simulink model "RHONN_EKF_FEEDBACK_FINAL_28_JULIO_2021"  (R2017b)
settings: Solver=ode1  StartTime=0.0  StopTime=60  FixedStep=0.001  RelTol=1e-3
model workspace (MATLAB code in the model file):
  | % ESTADOS INICIALES DE LOS ESTADOS X1, X2 Y X3
  | % Donde:
  | % x1 es representado con un vector de 3x1.
  | % x2 es representado con un vector de 2x1.
  | % x3 es representado con un vector de 2x1.
  | 
  | % Definir estados iniciales de las variables x11, x12 y x13 respectivamente.
  | init_x11 = 0;
  | init_x12 = 0;
  | init_x13 = 0;
  | % Estado inicial de x1
  | init_state_x1 = [init_x11; init_x12; init_x13];
  | 
  | % Definir estados iniciales de las variables x21 y x22 respectivamente.
  | init_x21 = 0.1;
  | init_x22 = 0.1;
  | % Estado inicial de x2
  | init_state_x2 = [init_x21; init_x22];
  | 
  | % Definir estados iniciales de las variables x31 y x32 respectivamente.
  | init_x31 = 0.1;
  | init_x32 = 0.1;
  | % Estado inicial de x3
  | init_state_x3 = [init_x31; init_x32];
  | 
  | % Definir el estado inicial de la ley de control U, representado por un vector de 2x1.
  | init_U1 = -1;
  | init_U2 = -1;
  | init_U = [init_U1; init_U2];
  | 
  | % INICIALIZACION DE VARIABLES >>>>>>>>>>>>>>>>>>>>>>>>>>>>>>>>
  | 
  |     %Constantes iniciales
  |     %La mitad del ancho del robot mobil.
  |     R = 0.75;
  |     %La distancia del centro de Pc del robot mobil a la mitad del punto medio
  |     %de P0 en medio de las ruedas izquierda y derecha.
  |     d = 0.3;
  |     %Radio de la rueda.
  |     r = 0.15;
  |     %Masa del cuerpo.
  |     mc = 30;
  |     %Masa de la rueda con motor.
  |     mw = 1;
  |     %Ic,Iw,Im son los momentos de inercia del cuerpo sobre el eje vertical a
  |     %traves de Pc.
  |     Ic = 15.625;
  |     Iw = 0.005;
  |     Im = 0.0025;
  |     %Resistencia.
  |     Ra = diag([2.5,2.5]);
  |     %Inductancia.
  |     La = diag([0.048,0.048]);
  |     %Coeficiente de fuera electromotriz trasero.
  |     KE = diag([0.02,0.02]);
  |     %Relacion de transmision.
  |     N = diag([62.55,62.55]);
  |     %Constante de torque del motor.
  |     KT = diag([0.2613,0.2613]);
  |     %d11, d12 son los coeficientes de amortiguamiento.
  |     d11 = 0.5;
  |     d12 = d11;
  |     %>>>>>>>>>>>>>>>>>>>>>>>>>>>>>>>>>>>>>>>>>>>>>>>>>>>>>>>><
  | 
  |     m = mc + (2 * mw);
  |     I = (mc * (d ^ 2)) + (2 * mw * (R^2)) + Ic + (2*Im);
  |     m11 = 0.25 * ( R ^ -2 ) * (r ^ 2) * ((m * (R ^ 2)) + I) + Iw;
  |     m12 = 0.25 * ( R ^ -2 ) * (r ^ 2) * ((m * (R ^ 2)) - I);
  |     M = [m11, m12; m12, m11];
  |     D = diag([d11, d12]);
  | 
  | 
  |  %VALORES HUERISTICOS SEGUN EL PAPER
  | %MODELO MATEMATICO
  | 
  | 
  | %Constantes iniciales
  | %La mitad del ancho del robot mobil.
  | R = 0.75;
  | %La distancia del centro de Pc del robot mobil a la mitad del punto medio
  | %de P0 en medio de las ruedas izquierda y derecha.
  | d = 0.3;
  | %Radio de la rueda.
  | r = 0.15;
  | %Masa del cuerpo.
  | mc = 30;
  | %Masa de la rueda con motor.
  | mw = 1;
  | %Ic,Iw,Im son los momentos de inercia del cuerpo sobre el eje vertical a
  | %traves de Pc.
  | Ic = 15.625;
  | Iw = 0.005;
  | Im = 0.0025;
  | %Resistencia.
  | Ra = diag([2.5,2.5]);
  | %Inductancia.
  | La = diag([0.048,0.048]);
  | %Coeficiente de fuera electromotriz trasero.
  | KE = diag([0.02,0.02]);
  | %Relacion de transmision.
  | N = diag([62.55,62.55]);
  | %Constante de torque del motor.
  | KT = diag([0.2613,0.2613]);
  | %d11, d12 son los coeficientes de amortiguamiento.
  | d11 = 0.5;
  | d12 = d11;
  | 
  | 
  | 
  | %NOTA : los valores cuya definicion se encuentre en minuscula
  | %se utiliza para generar de manera dinamica con programacion
  | %la variable final que se utiliza en el programa.
  | %De manera que si llegara a ser necesario solo se modificarian las variables iniciales
  | 
  | %VARIABLES INICIALES ========================================
  | 
  | p1 = 1 * (10^8);
  | p2 = 1 * (10^2);
  | p3 = 1 * (10^8);
  | p4 = 1 * (10^2);
  | p5 = 1 * (10^2);
  | p6 = 1 * (10^2);
  | p7 = 1 * (10^2);
  | 
  | r1 = 1 * (10^4);
  | r2 = 5 * (10^4);
  | r3 = 1 * (10^4);
  | r4 = 1 * (10^1);
  | r5 = 1 * (10^1);
  | r6 = 1 * (10^3);
  | r7 = 1 * (10^3);
  | 
  | q1 = 5 * (10^5);
  | q2 = 5 * (10^5);
  | q3 = 5 * (10^5);
  | q4 = 1 * (10^1);
  | q5 = 1 * (10^1);
  | q6 = 1 * (10^3);
  | q7 = 1 * (10^3);
  | 
  | G1 = 0.00001;
  | G2 = 0.00001;
  | 
  | %VALOREES INICIALES DE LOS PESOS USADOS EN EKF
  | 
  | %PESOS DE W1
  | W11 = 0.1;
  | W12 = 0.1;
  | %PESOS DE W2
  | W21 = 0.1;
  | W22 = 0.1;
  | %PESOS DE W3
  | W31 = 0.1;
  | W32 = 0.1;
  | %PESOS DE W4
  | W41 = 0.1;
  | W42 = 0.1;
  | W43 = 0.1;
  | W44 = 0.1;
  | %PESOS DE W5
  | W51 = 0.1;
  | W52 = 0.1;
  | W53 = 0.1;
  | W54 = 0.1;
  | %PESOS DE W6
  | W61 = 0.1;
  | W62 = 0.1;
  | W63 = 0.1;
  | W64 = 0.1;
  | %PESOS DE W7
  | W71 = 0.1;
  | W72 = 0.1;
  | W73 = 0.1;
  | W74 = 0.1;
  | 
  | %VALOR DE LAS SIGMOIDALES SUAVES
  | B = 2 * exp(-3);    %Este valor debe ser mayor a cero pero en base a mis observaciones menor a 1.
  | FO = 1;   %Este valor es obtenido de la tesis de la Dra Alma debe ser CERCANO y MENOR a 1, si este se vuelve 1 funcionara como FKE unicamente
  | 
  | 
  | %VARIABLES FINALES ========================================
  | 
  | %PARAMETROS DE ENTRENAMIENTO EKF PARA RHONN 1
  | W1 = [W11; W12]; %VALOR INICIAL de Vector de pesos para x1
  | P1 = diag([p1, p1]); %VALOR INICIAL de Matriz diagonal inicial de P1
  | R1 = r1; % Valor de R1
  | Q1 = diag([q1, q1]); % Valor de Q1
  | 
  | %PARAMETROS DE ENTRENAMIENTO EKF PARA RHONN 2
  | W2 = [W21; W22]; %VALOR INICIAL de Vector de pesos para x2
  | P2 = diag([p2, p2]); %VALOR INICIAL de Matriz diagonal inicial de P2
  | R2 = r2; % Valor de R2
  | Q2 = diag([q2, q2]); % Valor de Q2
  | 
  | %PARAMETROS DE ENTRENAMIENTO EKF PARA RHONN 3
  | W3 = [W31; W32]; %VALOR INICIAL de Vector de pesos para x3
  | P3 = diag([p3, p3]); %VALOR INICIAL de Matriz diagonal inicial de P3
  | R3 = r3; % Valor de R3
  | Q3 = diag([q3, q3]); % Valor de Q3
  | 
  | %PARAMETROS DE ENTRENAMIENTO EKF PARA RHONN 4
  | W4 = [W41; W42; W43; W44]; %VALOR INICIAL de Vector de pesos para x4
  | P4 = diag([p4, p4, p4, p4]); %VALOR INICIAL de Matriz diagonal inicial de P4
  | R4 = r4; % Valor de R4
  | Q4 = diag([q4, q4, q4, q4]); % Valor de Q4
  | 
  | %PARAMETROS DE ENTRENAMIENTO EKF PARA RHONN 5
  | W5 = [W51; W52; W53; W54]; %VALOR INICIAL de Vector de pesos para x5
  | P5 = diag([p5, p5, p5, p5]); %VALOR INICIAL de Matriz diagonal inicial de P5
  | R5 = r5; % Valor de R5
  | Q5 = diag([q5, q5, q5, q5]); % Valor de Q5
  | 
  | %PARAMETROS DE ENTRENAMIENTO EKF PARA RHONN 6
  | W6 = [W61; W62; W63; W64]; %VALOR INICIAL de Vector de pesos para x6
  | P6 = diag([p6, p6, p6, p6]); %VALOR INICIAL de Matriz diagonal inicial de P6
  | R6 = r6; % Valor de R6
  | Q6 = diag([q6, q6, q6, q6]); % Valor de Q6
  | 
  | %PARAMETROS DE ENTRENAMIENTO EKF PARA RHONN 7
  | W7 = [W71; W72; W73; W74]; %VALOR INICIAL de Vector de pesos para x7
  | P7 = diag([p7, p7, p7, p7]); %VALOR INICIAL de Matriz diagonal inicial de P7
  | R7 = r7; % Valor de R7
  | Q7 = diag([q7, q7, q7, q7]); % Valor de Q7
  | 
  | 
  | % PARAMETROS DEL CONTROL POR RETROALIMENTACION
  | % Donde K1 es representado con una matriz diagonal 3x3
  | % Donde K2 es representado con una matriz diagonal 2x2
  | % Donde K3 es representado con una matriz diagonal 2x2
  | 
  | % Ganancias individuales de la diagonal K1
  | k11 = 70;
  | k12 = k11;
  | k13 = k11;
  | 
  | % Ganancias individuales de la diagonal K2.
  | k21 = 50;
  | k22 = k21;
  | 
  | % Ganancias individuales de la diagonal K3.
  | k31 = 200;
  | k32 = k31;
  | 
  | % Matrices de gananciasK1, K2, K3.
  | K1 = diag([k11, k12, k13]);
  | K2 = diag([k21, k22]);
  | K3 = diag([k31, k32]);
libraries: simulink x5
(part 2 of 2)

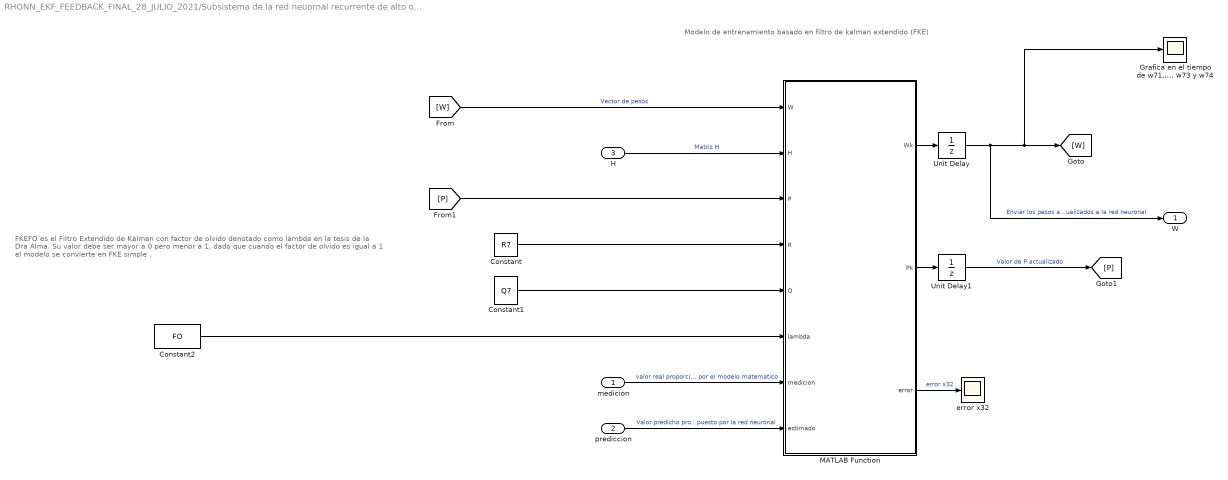
== system RHONN_EKF_FEEDBACK_FINAL_28_JULIO_2021/Subsistema de la red neuornal recurrente de alto orden (RHONN)/X7_RHONN/X7_EKF ==
  note: FKEFO es el Filtro Extendido de Kalman con factor de olvido
      |
      | denotado como lambda en la tesis de la Dra Alma.
      | Su valor debe ser mayor a 0 pero menor a 1, dado que cuando
      | el factor de olvido es igual a 1 el modelo se convierte en FKE simple .
  note: Modelo de entrenamiento basado en filtro de kalman extendido (FKE)
  medicion : Inport
  prediccion : Inport  Port=2
  H : Inport  Port=3
  Constant : Constant  Value=R7
  Constant1 : Constant  Value=Q7
  Constant2 : Constant  Value=FO
  "Grafica en el tiempo de w71, w72, w73 y w74" : Scope
  MATLAB Function : MATLAB Function  TreatAsAtomicUnit=on
  Unit Delay : UnitDelay  InitialCondition=W7  SampleTime=-1
  Unit Delay1 : UnitDelay  InitialCondition=P7  SampleTime=-1
  error x32 : Scope
  W : Outport
  wires:
  prediccion/1 -> MATLAB Function/8(estimado)  "Valor predicho propuesto por la red neuronal"
  medicion/1 -> MATLAB Function/7(medicion)  "valor real proporcionado por el modelo matematico"
  MATLAB Function/1(Wk) -> Unit Delay/1
  [W] -> MATLAB Function/1(W)  "Vector de pesos"
  MATLAB Function/2(Pk) -> Unit Delay1/1
  [P] -> MATLAB Function/3(P)
  Constant/1 -> MATLAB Function/4(R)
  Constant1/1 -> MATLAB Function/5(Q)
  H/1 -> MATLAB Function/2(H)  "Matriz H"
  Unit Delay1/1 -> [P]  "Valor de P actualizado"
  Unit Delay/1 -> "Grafica en el tiempo de w71, w72, w73 y w74"/1, [W], W/1  "Enviar los pesos actualizados a la red neuronal"
  Constant2/1 -> MATLAB Function/6(lambda)
  MATLAB Function/3(error) -> error x32/1  "error x32"

== matlab function RHONN_EKF_FEEDBACK_FINAL_28_JULIO_2021/Subsistema del robot no-holonomico, Modelo cinematico/NonHolonomic robot PLANT Function ==
  data: x11 input; dx1 output; x12 input; x13 input; dx13 input; x21 input; x22 input; x31 input; x32 input; Td1 input; Td2 input; dx2 output; dx3 output; u input
function [dx1,dx2,dx3]  = ROBOT(x11, x12, x13, dx13, x21, x22, x31, x32, Td1, Td2, u)
    
    %Definicion de las matrices de parametros del robot.(Entradas).
    x1 = [x11; x12; x13];
    x2 = [x21; x22];
    x3 = [x31; x32];
    
    %Vector de perturbaciones.
    Td = [Td1; Td2];
    
    %Vector de torques.
    %T = [T1; T2];
   
    %Vector de voltajes
    %u = [u1;u2];
    %Constantes iniciales
    %La mitad del ancho del robot mobil.
    R = 0.75;
    %La distancia del centro de Pc del robot mobil a la mitad del punto medio
    %de P0 en medio de las ruedas izquierda y derecha.
    d = 0.3;
    %Radio de la rueda.
    r = 0.15;
    %Masa del cuerpo.
    mc = 30;
    %Masa de la rueda con motor.
    mw = 1;
    %Ic,Iw,Im son los momentos de inercia del cuerpo sobre el eje vertical a
    %traves de Pc.
    Ic = 15.625;
    Iw = 0.005;
    Im = 0.0025;
    %Resistencia.
    Ra = diag([2.5,2.5]);
    %Inductancia.
    La = diag([0.048,0.048]);
    %Coeficiente de fuera electromotriz trasero.
    KE = diag([0.02,0.02]);
    %Relacion de transmision.
    N = diag([62.55,62.55]);
    %Constante de torque del motor.
    KT = diag([0.2613,0.2613]);
    %d11, d12 son los coeficientes de amortiguamiento.
    d11 = 0.5;
    d12 = d11;

    %%%%%%%%%%%%%% Constantes productos de otras constantes%%%%%%%%%%%%%%%%%%%%

    %Matriz cinematica del robot
    Jx1 = 0.5*r*[cos(x13), cos(x13); sin(x13), sin(x13); 1/R,-1/R];
    
    m = mc + (2 * mw);
    I = (mc * (d ^ 2)) + (2 * mw * (R^2)) + Ic + (2*Im);
    m11 = 0.25 * ( R ^ -2 ) * (r ^ 2) * ((m * (R ^ 2)) + I) + Iw;
    m12 = 0.25 * ( R ^ -2 ) * (r ^ 2) * ((m * (R ^ 2)) - I);
    M = [m11, m12; m12, m11];
    D = diag([d11, d12]);
    Cdx1 = 0.5*(1/R)*(r^2)*mc*d*[0, dx13; -dx13 0];
    
    %Definiendo las salidas de la funcion 
    dx1 = Jx1*x2;
    dx2=M\(-Cdx1*x2-D*x2-Td+(N*KT*x3));
    dx3 = La\(u-Ra*x3-(N*KE*x2));
    
    
end

== matlab function RHONN_EKF_FEEDBACK_FINAL_28_JULIO_2021/Trayectoria de referencia generada/Reference robot function ==
  data: Vr input; Wr input; dx1r output; Or input
function dx1r = fcn(Vr,Wr,Or)
    %   Definimos la señal de entrada que viene en el vector Zr' 
    dor = Wr;
    dxr = Vr * cos(Or);
    dyr = Vr * sin(Or);
    dx1r = [dxr; dyr; dor];

== matlab function RHONN_EKF_FEEDBACK_FINAL_28_JULIO_2021/Subsistema de la red neuornal recurrente de alto orden (RHONN)/X1_RHONN/Sigmoidal suave1/Sigmoidal suave ==
  data: B input; sig output; c input
function sig = fcn(B, c)

%Ecuacion sigmoidal suave
sig = 1/ (1 + exp(-B * c));

== matlab function RHONN_EKF_FEEDBACK_FINAL_28_JULIO_2021/Subsistema de la red neuornal recurrente de alto orden (RHONN)/X1_RHONN/Sigmoidal suave3/Sigmoidal suave ==
  data: B input; sig output; c input
function sig = fcn(B, c)

%Ecuacion sigmoidal suave
sig = 1/ (1 + exp(-B * c));

== matlab function RHONN_EKF_FEEDBACK_FINAL_28_JULIO_2021/Subsistema de la red neuornal recurrente de alto orden (RHONN)/X1_RHONN/X1_RHONN ==
  data: W input; pred output; Sx11 input; Sx12 input
function pred = fcn(W,Sx11,Sx12)
    
    %Pesos de la RHONN
    w11 = W(1);
    w12 = W(2);
    %Ecuacion de prediccion
    pred = ( w11 * Sx11 ) + ( w12 * Sx12 );

== matlab function RHONN_EKF_FEEDBACK_FINAL_28_JULIO_2021/Subsistema de control por retroalimentacion/MATLAB Function ==
  data: x1 input; x1r input; x2 input; dx1r input; x13 input; dx13 input; e1 output; e2 output; e3 output; U output; x3 input; k1 input; k2 input; k3 input
function [e1, e2, e3,U] = fcn(x1, x1r, x2,dx1r, x13, dx13, x3, k1, k2, k3)

   
    Td = [0.5; 0.5];
    %Constantes iniciales
    R = 0.75;    %La mitad del ancho del robot mobil.
    d = 0.3; %La distancia del centro de Pc del robot mobil a la mitad del punto medio
             %de P0 en medio de las ruedas izquierda y derecha
    r = 0.15; %Radio de la rueda.
    mc = 30;  %Masa del cuerpo.
    mw = 1;  %Masa de la rueda con motor.
    %Ic,Iw,Im son los momentos de inercia del cuerpo sobre el eje vertical a
    %traves de Pc.
    Ic = 15.625;
    Iw = 0.005;
    Im = 0.0025;
   
    Ra = diag([2.5,2.5]);       %Resistencia.
    La = diag([0.048,0.048]);    %Inductancia.
    KE = diag([0.02,0.02]);     %Coeficiente de fuera electromotriz trasero.
    N = diag([62.55,62.55]);     %Relacion de transmision.
    KT = diag([0.2613,0.2613]);  %Constante de torque del motor.
    d11 = 0.5;         %d11, d12 son los coeficientes de amortiguamiento.
    d12 = d11;

    m = mc + (2 * mw);
    I = (mc * (d ^ 2)) + (2 * mw * (R^2)) + Ic + (2*Im);
    m11 = 0.25 * ( R ^ -2 ) * (r ^ 2) * ((m * (R ^ 2)) + I) + Iw;
    m12 = 0.25 * ( R ^ -2 ) * (r ^ 2) * ((m * (R ^ 2)) - I);
    M = [m11, m12; m12, m11];
    D = diag([d11, d12]);
    Cdx1 = 0.5 * (1/R) * (r ^ 2) * mc * d * [0, dx13; -dx13 0];
    
    %%%%%%%%%%%%%%%%%%%%%%%%%%%%%%%%%%%%%%%%%%%%%%%%%%%%%%%%%%%%%%%%%%%%%%%
    
    % Control
    %Matriz cinematica del robot
     
    Jx1=0.5*r*[cos(x13), cos(x13); sin(x13), sin(x13); 1/R,-1/R];
    Jx1_inversa = pinv(Jx1);
	%Control virtual para x2r virtual.
    e1=x1-x1r;
    x2r=Jx1_inversa*(-k1*e1-dx1r);
    e2=x2-x2r;
    % Control virtual para x3r virual.
    dx2r = diff(x2r);
    x3r = (N*KT)\(M*(-k2*e2+dx2r)+Cdx1*x2+D*x2+Td);
    e3=x3-x3r;
    % Control real U.
    dx3r = diff(x3r);
    U=La*(-k3*e3+dx3r)+Ra*x3+N*KE*x2;
end

== matlab function RHONN_EKF_FEEDBACK_FINAL_28_JULIO_2021/Subsistema de la red neuornal recurrente de alto orden (RHONN)/X1_RHONN/X1_EKF/MATLAB Function ==
  settings: updateMethod=DISCRETE
  data: W input; Wk output; H input; P input; R input; Q input; lambda input; medicion input; estimado input; Pk output; error output
function [Wk, Pk, error] = fcn(W, H, P, R, Q, lambda, medicion, estimado)
    % Se inicializan las dimenciones de las variables K y M para evitar
    % error de dimensiones al momento de compilar.
    persistent K
    persistent M
    
    if isempty(K)
        K = zeros(2,1);
    end
    
    if isempty(M)
        M = zeros(1,1);
    end
    
    % NOTA: Para este caso
    % W, H, P, R, Q representan los valores en k_esima
    % Wk, Pk representan los valores de k + 1
    
    %L es el numero total de pesos = 2 (w11,w12)
    %m es el numero de salidas = 1 (X(k+1))
    
    %P es una matriz L x L (2x2)
    %R es una matriz m x m (1x1)
    %Q es una matriz L x L (2x2)
    %K es una matriz L x m (2x1)
    
    %lambda es el factor de olvido si lambda = 1 el modelo deja de ser
    %FKEFO y se vuelve FKE
    error = medicion - estimado;
    %Mi(k)
    M = (R * lambda ) + (H * P * H');
    %K(k)
    K = (P * H' )/(M);
    %W(k+1)
    Wk = W + K * (medicion - estimado);
    %P(k+1)
    Pk = (P * (1/lambda)) - ((1/lambda) * K * H * P) + Q;

== matlab function RHONN_EKF_FEEDBACK_FINAL_28_JULIO_2021/Subsistema de la red neuornal recurrente de alto orden (RHONN)/X1_RHONN/Generador de matriz H ==
  data: Sx11 input; H output; Sx12 input
function H = generador_H(Sx11,Sx12)
    %Matrix H para H1 dado 
    %Esta matriz ha sido generada con respecto a la ecuacion 14
    H = [Sx11,Sx12];

== matlab function RHONN_EKF_FEEDBACK_FINAL_28_JULIO_2021/Subsistema de la red neuornal recurrente de alto orden (RHONN)/X2_RHONN/Generador de matriz H ==
  data: Sx11 input; H output; Sx12 input
function H = generador_H(Sx11,Sx12)
    %Matrix H para H1 dado 
    %Esta matriz ha sido generada con respecto a la ecuacion 14
    %MAS INFORMACION EN LA OBTENCION DE LA MATRIZ H PARA CADA ESTADO
    % https://github.com/alfredoaguiararce/robot-uniciclo-python/blob/main/Demostracion_de_matrices_H.ipynb
   
    H = [Sx11,Sx12];

== matlab function RHONN_EKF_FEEDBACK_FINAL_28_JULIO_2021/Subsistema de la red neuornal recurrente de alto orden (RHONN)/X2_RHONN/Sigmoidal suave1/Sigmoidal suave ==
  data: B input; sig output; c input
function sig = fcn(B, c)

%Ecuacion sigmoidal suave
sig = 1/ (1 + exp(-B * c));

== matlab function RHONN_EKF_FEEDBACK_FINAL_28_JULIO_2021/Subsistema de la red neuornal recurrente de alto orden (RHONN)/X2_RHONN/Sigmoidal suave3/Sigmoidal suave ==
  data: B input; sig output; c input
function sig = fcn(B, c)

%Ecuacion sigmoidal suave
sig = 1/ (1 + exp(-B * c));

== matlab function RHONN_EKF_FEEDBACK_FINAL_28_JULIO_2021/Subsistema de la red neuornal recurrente de alto orden (RHONN)/X2_RHONN/X2_EKF/MATLAB Function ==
  settings: updateMethod=DISCRETE
  data: W input; Wk output; H input; P input; R input; Q input; lambda input; medicion input; estimado input; Pk output; error output
function [Wk,Pk, error] = fcn(W, H, P, R, Q, lambda, medicion, estimado)
    % Se inicializan las dimenciones de las variables K y M para evitar
    % error de dimensiones al momento de compilar.
    persistent K
    persistent M
    
    if isempty(K)
        K = zeros(2,1);
    end
    
    if isempty(M)
        M = zeros(1,1);
    end
    
    % NOTA: Para este caso
    % W, H, P, R, Q representan los valores en k_esima
    % Wk, Pk representan los valores de k + 1
    
    %L es el numero total de pesos = 2 (w11,w12)
    %m es el numero de salidas = 1 (X(k+1))
    
    %P es una matriz L x L (2x2)
    %R es una matriz m x m (1x1)
    %Q es una matriz L x L (2x2)
    %K es una matriz L x m (2x1)
    
    %lambda es el factor de olvido si lambda = 1 el modelo deja de ser
    %FKEFO y se vuelve FKE
    
    error = medicion - estimado;
    %Mi(k)
    M = (R * lambda ) + (H * P * H');
    %K(k)
    K = (P * H' )/(M);
    %W(k+1)
    Wk = W + K * (medicion - estimado);
    %P(k+1)
    Pk = (P * (1/lambda)) - ((1/lambda) * K * H * P) + Q;

== matlab function RHONN_EKF_FEEDBACK_FINAL_28_JULIO_2021/Subsistema de la red neuornal recurrente de alto orden (RHONN)/X2_RHONN/X2_RHONN_function ==
  data: W input; pred output; Sx11 input; Sx12 input
function pred = fcn(W,Sx11,Sx12)

    %Pesos de X2
    w21 = W(1);
    w22 = W(2);
    %ecuacion de prediccion X2
    pred = ( w21 * Sx11 ) + ( w22 * Sx12 );

== matlab function RHONN_EKF_FEEDBACK_FINAL_28_JULIO_2021/Subsistema de la red neuornal recurrente de alto orden (RHONN)/X3_RHONN/Generador de matriz H ==
  data: Sx11 input; H output; Sx12 input
function H = generador_H(Sx11,Sx12)
    %Matrix H para H1 dado 
    %Esta matriz ha sido generada con respecto a la ecuacion 14
    %MAS INFORMACION EN LA OBTENCION DE LA MATRIZ H PARA CADA ESTADO
    % https://github.com/alfredoaguiararce/robot-uniciclo-python/blob/main/Demostracion_de_matrices_H.ipynb
   
    H = [Sx11,Sx12];

== matlab function RHONN_EKF_FEEDBACK_FINAL_28_JULIO_2021/Subsistema de la red neuornal recurrente de alto orden (RHONN)/X3_RHONN/Sigmoidal suave1/Sigmoidal suave ==
  data: B input; sig output; c input
function sig = fcn(B, c)

%Ecuacion sigmoidal suave
sig = 1/ (1 + exp(-B * c));

== matlab function RHONN_EKF_FEEDBACK_FINAL_28_JULIO_2021/Subsistema de la red neuornal recurrente de alto orden (RHONN)/X3_RHONN/Sigmoidal suave3/Sigmoidal suave ==
  data: B input; sig output; c input
function sig = fcn(B, c)

%Ecuacion sigmoidal suave
sig = 1/ (1 + exp(-B * c));

== matlab function RHONN_EKF_FEEDBACK_FINAL_28_JULIO_2021/Subsistema de la red neuornal recurrente de alto orden (RHONN)/X3_RHONN/X3_EKF/MATLAB Function ==
  settings: updateMethod=DISCRETE
  data: W input; Wk output; H input; P input; R input; Q input; lambda input; medicion input; estimado input; Pk output; error output
function [Wk,Pk, error] = fcn(W, H, P, R, Q, lambda, medicion, estimado)
    
    % Se inicializan las dimenciones de las variables K y M para evitar
    % error de dimensiones al momento de compilar.
    persistent K
    persistent M
    
    if isempty(K)
        K = zeros(4,1);
    end
    
    if isempty(M)
        M = zeros(1,1);
    end
    % NOTA: Para este caso
    % W, H, P, R, Q representan los valores en k_esima
    % Wk, Pk representan los valores de k + 1
    
    %L es el numero total de pesos = 2 (w11,w12)
    %m es el numero de salidas = 1 (X(k+1))
    
    %P es una matriz L x L (2x2)
    %R es una matriz m x m (1x1)
    %Q es una matriz L x L (2x2)
    %K es una matriz L x m (2x1)
    
    %lambda es el factor de olvido si lambda = 1 el modelo deja de ser
    %FKEFO y se vuelve FKE
    
    error = medicion - estimado;
    %Mi(k)
    M = (R * lambda ) + (H * P * H');
    %K(k)
    K = (P * H' )/(M);
    %W(k+1)
    Wk = W + K * (medicion - estimado);
    %P(k+1)
    Pk = (P * (1/lambda)) - ((1/lambda) * K * H * P) + Q;

== matlab function RHONN_EKF_FEEDBACK_FINAL_28_JULIO_2021/Subsistema de la red neuornal recurrente de alto orden (RHONN)/X3_RHONN/X3_RHONN_function ==
  data: W input; pred output; Sx11 input; Sx12 input
function pred = fcn(W,Sx11,Sx12)

    %Pesos de X3
    w31 = W(1);
    w32 = W(2);
    %ecuacion de prediccion X2
    pred = ( w31 * Sx11 ) + ( w32 * Sx12 );

== matlab function RHONN_EKF_FEEDBACK_FINAL_28_JULIO_2021/Subsistema de la red neuornal recurrente de alto orden (RHONN)/X4_RHONN/Generador de matriz H ==
  data: Sx11 input; H output; Sx12 input; Sx21 input; Sx31 input
function H = generador_H(Sx11,Sx12,Sx21,Sx31)
    %Matrix H para H1 dado 
    %Esta matriz ha sido generada con respecto a la ecuacion 14
    %MAS INFORMACION EN LA OBTENCION DE LA MATRIZ H PARA CADA ESTADO
    % https://github.com/alfredoaguiararce/robot-uniciclo-python/blob/main/Demostracion_de_matrices_H.ipynb
   
    H = [Sx11,Sx12,Sx21,Sx31];

== matlab function RHONN_EKF_FEEDBACK_FINAL_28_JULIO_2021/Subsistema de la red neuornal recurrente de alto orden (RHONN)/X4_RHONN/Sigmoidal suave1/Sigmoidal suave ==
  data: B input; sig output; c input
function sig = fcn(B, c)

%Ecuacion sigmoidal suave
sig = 1/ (1 + exp(-B * c));

== matlab function RHONN_EKF_FEEDBACK_FINAL_28_JULIO_2021/Subsistema de la red neuornal recurrente de alto orden (RHONN)/X4_RHONN/Sigmoidal suave3/Sigmoidal suave ==
  data: B input; sig output; c input
function sig = fcn(B, c)

%Ecuacion sigmoidal suave
sig = 1/ (1 + exp(-B * c));

== matlab function RHONN_EKF_FEEDBACK_FINAL_28_JULIO_2021/Subsistema de la red neuornal recurrente de alto orden (RHONN)/X4_RHONN/Sigmoidal suave2/Sigmoidal suave ==
  data: B input; sig output; c input
function sig = fcn(B, c)

%Ecuacion sigmoidal suave
sig = 1/ (1 + exp(-B * c));

== matlab function RHONN_EKF_FEEDBACK_FINAL_28_JULIO_2021/Subsistema de la red neuornal recurrente de alto orden (RHONN)/X4_RHONN/Sigmoidal suave4/Sigmoidal suave ==
  data: B input; sig output; c input
function sig = fcn(B, c)

%Ecuacion sigmoidal suave
sig = 1/ (1 + exp(-B * c));

== matlab function RHONN_EKF_FEEDBACK_FINAL_28_JULIO_2021/Subsistema de la red neuornal recurrente de alto orden (RHONN)/X4_RHONN/X4_EKF/MATLAB Function ==
  settings: updateMethod=DISCRETE
  data: W input; Wk output; H input; P input; R input; Q input; lambda input; medicion input; estimado input; Pk output; error output
function [Wk,Pk, error] = fcn(W, H, P, R, Q, lambda, medicion, estimado)
    
    % Se inicializan las dimenciones de las variables K y M para evitar
    % error de dimensiones al momento de compilar.
    persistent K
    persistent M
    
    if isempty(K)
        K = zeros(4,1);
    end
    
    if isempty(M)
        M = zeros(1,1);
    end
    
    % NOTA: Para este caso
    % W, H, P, R, Q representan los valores en k_esima
    % Wk, Pk representan los valores de k + 1
    
    %L es el numero total de pesos = 2 (w11,w12)
    %m es el numero de salidas = 1 (X(k+1))
    
    %P es una matriz L x L (2x2)
    %R es una matriz m x m (1x1)
    %Q es una matriz L x L (2x2)
    %K es una matriz L x m (2x1)
    
    %lambda es el factor de olvido si lambda = 1 el modelo deja de ser
    %FKEFO y se vuelve FKE
    error = medicion - estimado;
    %Mi(k)
    M = (R * lambda ) + (H * P * H');
    %K(k)
    K = (P * H' )/(M);
    %W(k+1)
    Wk = W + K * (medicion - estimado);
    %P(k+1)
    Pk = (P * (1/lambda)) - ((1/lambda) * K * H * P) + Q;

== matlab function RHONN_EKF_FEEDBACK_FINAL_28_JULIO_2021/Subsistema de la red neuornal recurrente de alto orden (RHONN)/X4_RHONN/X4_RHONN_function ==
  data: W input; pred output; Sx11 input; Sx12 input; Sx21 input; Sx31 input
function pred = fcn(W,Sx11,Sx12, Sx21, Sx31)

    %Pesos de X3
    w41 = W(1);
    w42 = W(2);
    w43 = W(3);
    w44 = W(4);
    %ecuacion de prediccion X2
    pred = ( w41 * Sx11 ) + ( w42 * Sx12 )+ ( w43 * Sx21 )+ ( w44 * Sx31 );

== matlab function RHONN_EKF_FEEDBACK_FINAL_28_JULIO_2021/Subsistema de la red neuornal recurrente de alto orden (RHONN)/X5_RHONN/Generador de matriz H ==
  data: Sx11 input; H output; Sx12 input; Sx21 input; Sx31 input
function H = generador_H(Sx11,Sx12,Sx21,Sx31)
    %Matrix H para H1 dado 
    %Esta matriz ha sido generada con respecto a la ecuacion 14
    %MAS INFORMACION EN LA OBTENCION DE LA MATRIZ H PARA CADA ESTADO
    % https://github.com/alfredoaguiararce/robot-uniciclo-python/blob/main/Demostracion_de_matrices_H.ipynb
   
    H = [Sx11,Sx12,Sx21,Sx31];

== matlab function RHONN_EKF_FEEDBACK_FINAL_28_JULIO_2021/Subsistema de la red neuornal recurrente de alto orden (RHONN)/X5_RHONN/Sigmoidal suave1/Sigmoidal suave ==
  data: B input; sig output; c input
function sig = fcn(B, c)

%Ecuacion sigmoidal suave
sig = 1/ (1 + exp(-B * c));

== matlab function RHONN_EKF_FEEDBACK_FINAL_28_JULIO_2021/Subsistema de la red neuornal recurrente de alto orden (RHONN)/X5_RHONN/Sigmoidal suave2/Sigmoidal suave ==
  data: B input; sig output; c input
function sig = fcn(B, c)

%Ecuacion sigmoidal suave
sig = 1/ (1 + exp(-B * c));

== matlab function RHONN_EKF_FEEDBACK_FINAL_28_JULIO_2021/Subsistema de la red neuornal recurrente de alto orden (RHONN)/X5_RHONN/Sigmoidal suave3/Sigmoidal suave ==
  data: B input; sig output; c input
function sig = fcn(B, c)

%Ecuacion sigmoidal suave
sig = 1/ (1 + exp(-B * c));

== matlab function RHONN_EKF_FEEDBACK_FINAL_28_JULIO_2021/Subsistema de la red neuornal recurrente de alto orden (RHONN)/X5_RHONN/Sigmoidal suave4/Sigmoidal suave ==
  data: B input; sig output; c input
function sig = fcn(B, c)

%Ecuacion sigmoidal suave
sig = 1/ (1 + exp(-B * c));

== matlab function RHONN_EKF_FEEDBACK_FINAL_28_JULIO_2021/Subsistema de la red neuornal recurrente de alto orden (RHONN)/X5_RHONN/X5_EKF/MATLAB Function ==
  settings: updateMethod=DISCRETE
  data: W input; Wk output; H input; P input; R input; Q input; lambda input; medicion input; estimado input; Pk output; error output
function [Wk,Pk, error] = fcn(W, H, P, R, Q, lambda, medicion, estimado)
    
    % Se inicializan las dimenciones de las variables K y M para evitar
    % error de dimensiones al momento de compilar.
    persistent K
    persistent M
    
    if isempty(K)
        K = zeros(4,1);
    end
    
    if isempty(M)
        M = zeros(1,1);
    end
    
    % NOTA: Para este caso
    % W, H, P, R, Q representan los valores en k_esima
    % Wk, Pk representan los valores de k + 1
    
    %L es el numero total de pesos = 2 (w11,w12)
    %m es el numero de salidas = 1 (X(k+1))
    
    %P es una matriz L x L (2x2)
    %R es una matriz m x m (1x1)
    %Q es una matriz L x L (2x2)
    %K es una matriz L x m (2x1)
    
    %lambda es el factor de olvido si lambda = 1 el modelo deja de ser
    %FKEFO y se vuelve FKE
    error = medicion - estimado;
    
    %Mi(k)
    M = (R * lambda ) + (H * P * H');
    
    %K(k)
    K = (P * H' )/(M);
    
    %W(k+1)
    Wk = W + K * (medicion - estimado);
    %P(k+1)
    Pk = (P * (1/lambda)) - ((1/lambda) * K * H * P) + Q;

== matlab function RHONN_EKF_FEEDBACK_FINAL_28_JULIO_2021/Subsistema de la red neuornal recurrente de alto orden (RHONN)/X5_RHONN/X5_RHONN_function ==
  data: W input; pred output; Sx11 input; Sx12 input; Sx21 input; Sx31 input; G1 input; U1 input
function pred = fcn(W,Sx11,Sx12, Sx21, Sx31, G1, U1)

    %Pesos de X3
    w51 = W(1);
    w52 = W(2);
    w53 = W(3);
    w54 = W(4);
    %ecuacion de prediccion X2
    pred = ( w51 * Sx11 ) + ( w52 * Sx12 )+ ( w53 * Sx21 )+ ( w54 * Sx31 )+ (G1*U1);

== matlab function RHONN_EKF_FEEDBACK_FINAL_28_JULIO_2021/Subsistema de la red neuornal recurrente de alto orden (RHONN)/X6_RHONN/Generador de matriz H ==
  data: Sx11 input; H output; Sx12 input; Sx22 input; Sx32 input
function H = generador_H(Sx11,Sx12,Sx22,Sx32)
    %Matrix H para H1 dado 
    %Esta matriz ha sido generada con respecto a la ecuacion 14
    %MAS INFORMACION EN LA OBTENCION DE LA MATRIZ H PARA CADA ESTADO
    % https://github.com/alfredoaguiararce/robot-uniciclo-python/blob/main/Demostracion_de_matrices_H.ipynb
   
    H = [Sx11,Sx12,Sx22,Sx32];

== matlab function RHONN_EKF_FEEDBACK_FINAL_28_JULIO_2021/Subsistema de la red neuornal recurrente de alto orden (RHONN)/X6_RHONN/Sigmoidal suave1/Sigmoidal suave ==
  data: B input; sig output; c input
function sig = fcn(B, c)

%Ecuacion sigmoidal suave
sig = 1/ (1 + exp(-B * c));

== matlab function RHONN_EKF_FEEDBACK_FINAL_28_JULIO_2021/Subsistema de la red neuornal recurrente de alto orden (RHONN)/X6_RHONN/Sigmoidal suave2/Sigmoidal suave ==
  data: B input; sig output; c input
function sig = fcn(B, c)

%Ecuacion sigmoidal suave
sig = 1/ (1 + exp(-B * c));

== matlab function RHONN_EKF_FEEDBACK_FINAL_28_JULIO_2021/Subsistema de la red neuornal recurrente de alto orden (RHONN)/X6_RHONN/Sigmoidal suave3/Sigmoidal suave ==
  data: B input; sig output; c input
function sig = fcn(B, c)

%Ecuacion sigmoidal suave
sig = 1/ (1 + exp(-B * c));

== matlab function RHONN_EKF_FEEDBACK_FINAL_28_JULIO_2021/Subsistema de la red neuornal recurrente de alto orden (RHONN)/X6_RHONN/Sigmoidal suave4/Sigmoidal suave ==
  data: B input; sig output; c input
function sig = fcn(B, c)

%Ecuacion sigmoidal suave
sig = 1/ (1 + exp(-B * c));

== matlab function RHONN_EKF_FEEDBACK_FINAL_28_JULIO_2021/Subsistema de la red neuornal recurrente de alto orden (RHONN)/X6_RHONN/X6_EKF/MATLAB Function ==
  settings: updateMethod=DISCRETE
  data: W input; Wk output; H input; P input; R input; Q input; lambda input; medicion input; estimado input; Pk output; error output
function [Wk,Pk, error] = fcn(W, H, P, R, Q, lambda, medicion, estimado)
    % Se inicializan las dimenciones de las variables K y M para evitar
    % error de dimensiones al momento de compilar.
    persistent K
    persistent M
    
    if isempty(K)
        K = zeros(4,1);
    end
    
    if isempty(M)
        M = zeros(1,1);
    end
    % NOTA: Para este caso
    % W, H, P, R, Q representan los valores en k_esima
    % Wk, Pk representan los valores de k + 1
    
    %L es el numero total de pesos = 2 (w11,w12)
    %m es el numero de salidas = 1 (X(k+1))
    
    %P es una matriz L x L (2x2)
    %R es una matriz m x m (1x1)
    %Q es una matriz L x L (2x2)
    %K es una matriz L x m (2x1)
    
    %lambda es el factor de olvido si lambda = 1 el modelo deja de ser
    %FKEFO y se vuelve FKE
    error = medicion - estimado;
    %Mi(k)
    M = (R * lambda ) + (H * P * H');
    %K(k)
    K = (P * H' )/(M);
    %W(k+1)
    Wk = W + K * (medicion - estimado);
    %P(k+1)
    Pk = (P * (1/lambda)) - ((1/lambda) * K * H * P) + Q;

== matlab function RHONN_EKF_FEEDBACK_FINAL_28_JULIO_2021/Subsistema de la red neuornal recurrente de alto orden (RHONN)/X6_RHONN/X6_RHONN_function ==
  data: W input; pred output; Sx11 input; Sx12 input; Sx22 input; Sx32 input
function pred = fcn(W,Sx11,Sx12, Sx22, Sx32)

    %Pesos de X
    w61 = W(1);
    w62 = W(2);
    w63 = W(3);
    w64 = W(4);
    %ecuacion de prediccion X
    pred = ( w61 * Sx11 ) + ( w62 * Sx12 )+ ( w63 * Sx22 )+ ( w64 * Sx32 );

== matlab function RHONN_EKF_FEEDBACK_FINAL_28_JULIO_2021/Subsistema de la red neuornal recurrente de alto orden (RHONN)/X7_RHONN/Generador de matriz H ==
  data: Sx11 input; H output; Sx12 input; Sx22 input; Sx32 input
function H = generador_H(Sx11,Sx12,Sx22,Sx32)
    %Matrix H para H1 dado 
    %Esta matriz ha sido generada con respecto a la ecuacion 14
    %MAS INFORMACION EN LA OBTENCION DE LA MATRIZ H PARA CADA ESTADO
    % https://github.com/alfredoaguiararce/robot-uniciclo-python/blob/main/Demostracion_de_matrices_H.ipynb
   
    H = [Sx11,Sx12,Sx22,Sx32];

== matlab function RHONN_EKF_FEEDBACK_FINAL_28_JULIO_2021/Subsistema de la red neuornal recurrente de alto orden (RHONN)/X7_RHONN/Sigmoidal suave1/Sigmoidal suave ==
  data: B input; sig output; c input
function sig = fcn(B, c)

%Ecuacion sigmoidal suave
sig = 1/ (1 + exp(-B * c));

== matlab function RHONN_EKF_FEEDBACK_FINAL_28_JULIO_2021/Subsistema de la red neuornal recurrente de alto orden (RHONN)/X7_RHONN/Sigmoidal suave2/Sigmoidal suave ==
  data: B input; sig output; c input
function sig = fcn(B, c)

%Ecuacion sigmoidal suave
sig = 1/ (1 + exp(-B * c));

== matlab function RHONN_EKF_FEEDBACK_FINAL_28_JULIO_2021/Subsistema de la red neuornal recurrente de alto orden (RHONN)/X7_RHONN/Sigmoidal suave3/Sigmoidal suave ==
  data: B input; sig output; c input
function sig = fcn(B, c)

%Ecuacion sigmoidal suave
sig = 1/ (1 + exp(-B * c));

== matlab function RHONN_EKF_FEEDBACK_FINAL_28_JULIO_2021/Subsistema de la red neuornal recurrente de alto orden (RHONN)/X7_RHONN/Sigmoidal suave4/Sigmoidal suave ==
  data: B input; sig output; c input
function sig = fcn(B, c)

%Ecuacion sigmoidal suave
sig = 1/ (1 + exp(-B * c));

== matlab function RHONN_EKF_FEEDBACK_FINAL_28_JULIO_2021/Subsistema de la red neuornal recurrente de alto orden (RHONN)/X7_RHONN/X7_EKF/MATLAB Function ==
  settings: updateMethod=DISCRETE
  data: W input; Wk output; H input; P input; R input; Q input; lambda input; medicion input; estimado input; Pk output; error output
function [Wk,Pk, error] = fcn(W, H, P, R, Q, lambda, medicion, estimado)
    
    % Se inicializan las dimenciones de las variables K y M para evitar
    % error de dimensiones al momento de compilar.
    persistent K
    persistent M
    
    if isempty(K)
        K = zeros(4,1);
    end
    
    if isempty(M)
        M = zeros(1,1);
    end
    
    % NOTA: Para este caso
    % W, H, P, R, Q representan los valores en k_esima
    % Wk, Pk representan los valores de k + 1
    
    %L es el numero total de pesos = 2 (w11,w12)
    %m es el numero de salidas = 1 (X(k+1))
    
    %P es una matriz L x L (2x2)
    %R es una matriz m x m (1x1)
    %Q es una matriz L x L (2x2)
    %K es una matriz L x m (2x1)
    
    %lambda es el factor de olvido si lambda = 1 el modelo deja de ser
    %FKEFO y se vuelve FKE
    error =  medicion - estimado;
    %Mi(k)
    M = (R * lambda ) + (H * P * H');
    %K(k)
    K = (P * H' )/(M);
    %W(k+1)
    Wk = W + K * (medicion - estimado);
    %P(k+1)
    Pk = (P * (1/lambda)) - ((1/lambda) * K * H * P) + Q;

== matlab function RHONN_EKF_FEEDBACK_FINAL_28_JULIO_2021/Subsistema de la red neuornal recurrente de alto orden (RHONN)/X7_RHONN/X7_RHONN_function ==
  data: W input; pred output; Sx11 input; Sx12 input; Sx22 input; Sx32 input; G2 input; U2 input
function pred = fcn(W,Sx11,Sx12, Sx22, Sx32, G2, U2)

    %Pesos de X
    w71 = W(1);
    w72 = W(2);
    w73 = W(3);
    w74 = W(4);
    %ecuacion de prediccion X
    pred = ( w71 * Sx11 ) + ( w72 * Sx12 )+ ( w73 * Sx22 )+ ( w74 * Sx32 )+(G2*U2);
